simulink model "ass_1"  (R2020a)
settings: Solver=FixedStepAuto  StartTime=0.0  StopTime=10.0  FixedStep=1e-3  RelTol=1e-3  EnableMultiTasking=on
undefined symbols (not defined in the file): D0, D1, D10, D11, D12, D13, D2, D3, D4, D5, D6, D7, D8, D9, PTA0, PTA1, PTA2, PTB23, PTB9, PTC16, PTC17, PTC2, PTC3, PTC4, PTD0, PTD1, PTD2, PTD3
libraries: frdmk64flib x15
settings Model: ExtModeTrigDuration=5  Creator=wxavi  LastModifiedBy=wxavi
settings OptimizationCC: EnhancedBackFolding=on  PassReuseOutputArgsAs=Individual arguments  ZeroExternalMemoryAtStartup=off  ZeroInternalMemoryAtStartup=off  MaxStackSize=64  OptimizeBlockOrder=speed  DifferentSizesBufferReuse=on  OptimizationCustomize=off  EfficientTunableParamExpr=on
settings DebuggingCC: ParameterTunabilityLossMsg=error
settings HardwareCC: ProdBitPerPointer=32  ProdBitPerSizeT=32  ProdBitPerPtrDiffT=32  ProdLargestAtomicInteger=Long  ProdLargestAtomicFloat=Double  ProdWordSize=32  ProdHWDeviceType=ARM Compatible->ARM Cortex
settings SFSimCC: MATLABDynamicMemAlloc=off
settings RTWCC: SystemTargetFile=ert.tlc  HardwareBoard=NXP FRDM-K64F  TemplateMakefile=ert_default_tmf  Toolchain=GNU Tools for ARM Embedded Processors
settings CodeAppCC: ForceParamTrailComments=on  IgnoreCustomStorageClasses=off  OperatorAnnotations=on  SimulinkDataObjDesc=on  SFDataObjDesc=on  InsertBlockDesc=on

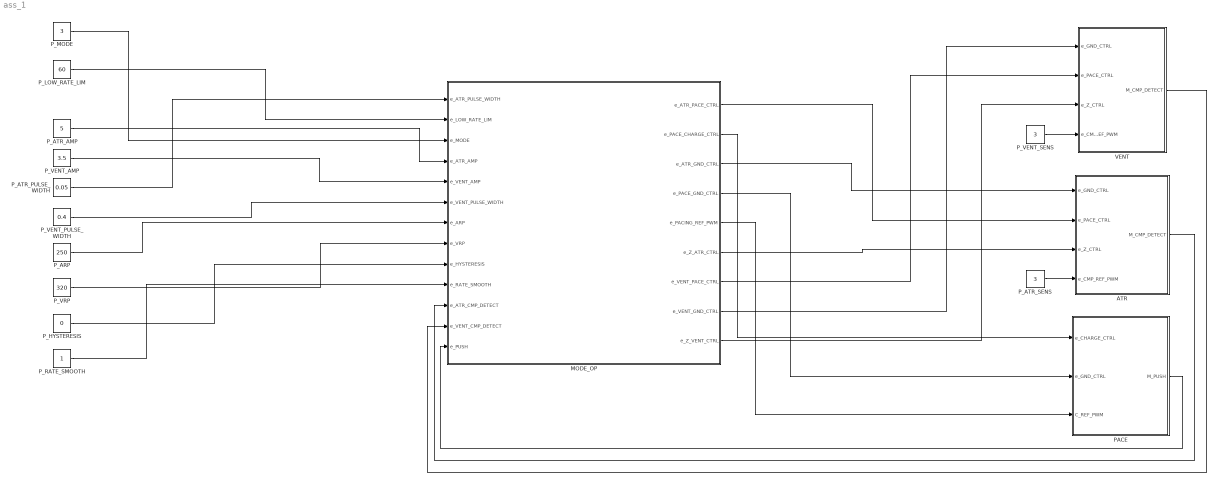
== system ass_1 ==
  ATR : Subsystem
  MODE_OP : Stateflow chart  TreatAsAtomicUnit=on
  PACE : Subsystem
  P_ARP : Constant  Value=250
  P_ATR_AMP : Constant  Value=5
  P_ATR_PULSE_WIDTH : Constant  Value=0.05
  P_ATR_SENS : Constant  Value=3
  P_HYSTERESIS : Constant  Value=0
  P_LOW_RATE_LIM : Constant  Value=60
  P_MODE : Constant  Value=3
  P_RATE_SMOOTH : Constant
  P_VENT_AMP : Constant  Value=3.5
  P_VENT_PULSE_WIDTH : Constant  Value=0.4
  P_VENT_SENS : Constant  Value=3
  P_VRP : Constant  Value=320
  VENT : Subsystem
  wires:
  P_LOW_RATE_LIM/1 -> MODE_OP/2(e_LOW_RATE_LIM)
  P_ATR_AMP/1 -> MODE_OP/4(e_ATR_AMP)
  P_VENT_AMP/1 -> MODE_OP/5(e_VENT_AMP)
  P_ATR_PULSE_WIDTH/1 -> MODE_OP/1(e_ATR_PULSE_WIDTH)
  P_VENT_PULSE_WIDTH/1 -> MODE_OP/6(e_VENT_PULSE_WIDTH)
  P_MODE/1 -> MODE_OP/3(e_MODE)
  P_ATR_SENS/1 -> ATR/4(e_CMP_REF_PWM)
  P_VENT_SENS/1 -> VENT/4(e_CMP_REF_PWM)
  P_ARP/1 -> MODE_OP/7(e_ARP)
  P_VRP/1 -> MODE_OP/8(e_VRP)
  P_HYSTERESIS/1 -> MODE_OP/9(e_HYSTERESIS)
  P_RATE_SMOOTH/1 -> MODE_OP/10(e_RATE_SMOOTH)
  ATR/1(M_CMP_DETECT) -> MODE_OP/11(e_ATR_CMP_DETECT)
  VENT/1(M_CMP_DETECT) -> MODE_OP/12(e_VENT_CMP_DETECT)
  PACE/1(M_PUSH) -> MODE_OP/13(e_PUSH)
  MODE_OP/1(e_ATR_PACE_CTRL) -> ATR/2(e_PACE_CTRL)
  MODE_OP/2(e_PACE_CHARGE_CTRL) -> PACE/1(e_CHARGE_CTRL)
  MODE_OP/3(e_ATR_GND_CTRL) -> ATR/1(e_GND_CTRL)
  MODE_OP/4(e_PACE_GND_CTRL) -> PACE/2(e_GND_CTRL)
  MODE_OP/5(e_PACING_REF_PWM) -> PACE/3(C_REF_PWM)
  MODE_OP/6(e_Z_ATR_CTRL) -> ATR/3(e_Z_CTRL)
  MODE_OP/7(e_VENT_PACE_CTRL) -> VENT/2(e_PACE_CTRL)
  MODE_OP/8(e_VENT_GND_CTRL) -> VENT/1(e_GND_CTRL)
  MODE_OP/9(e_Z_VENT_CTRL) -> VENT/3(e_Z_CTRL)

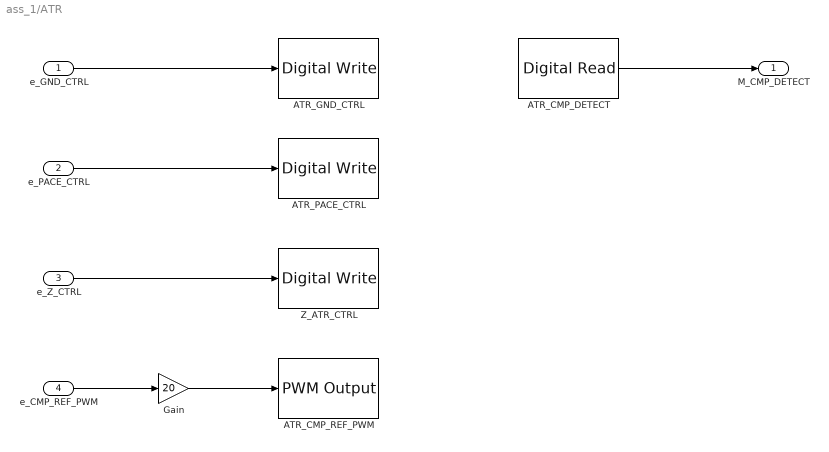
== system ass_1/ATR ==
  e_GND_CTRL : Inport
  e_PACE_CTRL : Inport  Port=2
  e_Z_CTRL : Inport  Port=3
  e_CMP_REF_PWM : Inport  Port=4
  ATR_CMP_DETECT : frdmk64flib/Digital Read  Whichpin=PTC16 (D0)  SampleTime=-1
  ATR_CMP_REF_PWM : frdmk64flib/PWM Output  Whichpin=PTC2 (D6)  InitialFrequency=2000  InitialDutyCycle=0
  ATR_GND_CTRL : frdmk64flib/Digital Write  Whichpin=PTD2 (D11)
  ATR_PACE_CTRL : frdmk64flib/Digital Write  Whichpin=PTA0 (D8)
  Gain : Gain  Gain=20
  Z_ATR_CTRL : frdmk64flib/Digital Write  Whichpin=PTB23 (D4)
  M_CMP_DETECT : Outport
  wires:
  e_Z_CTRL/1 -> Z_ATR_CTRL/1
  e_GND_CTRL/1 -> ATR_GND_CTRL/1
  e_PACE_CTRL/1 -> ATR_PACE_CTRL/1
  e_CMP_REF_PWM/1 -> Gain/1
  ATR_CMP_DETECT/1 -> M_CMP_DETECT/1
  Gain/1 -> ATR_CMP_REF_PWM/1

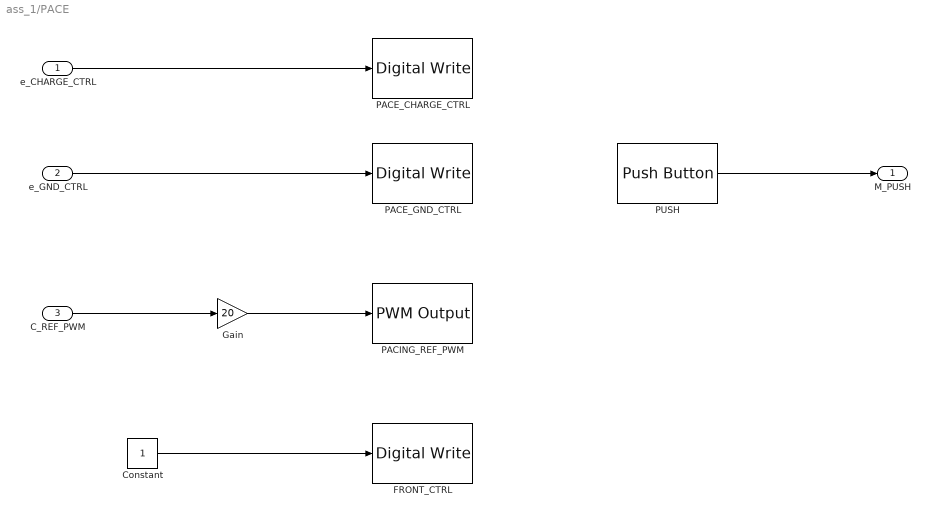
== system ass_1/PACE ==
  e_CHARGE_CTRL : Inport
  e_GND_CTRL : Inport  Port=2
  C_REF_PWM : Inport  Port=3
  Constant : Constant
  FRONT_CTRL : frdmk64flib/Digital Write  Whichpin=PTD1 (D13)
  Gain : Gain  Gain=20
  PACE_CHARGE_CTRL : frdmk64flib/Digital Write  Whichpin=PTB9 (D2)
  PACE_GND_CTRL : frdmk64flib/Digital Write  Whichpin=PTD0 (D10)
  PACING_REF_PWM : frdmk64flib/PWM Output  Whichpin=PTA2 (D5)  InitialFrequency=2000  InitialDutyCycle=0
  PUSH : frdmk64flib/Push Button  Whichswitch=SW2  SampleTime1=-1
  M_PUSH : Outport
  wires:
  Gain/1 -> PACING_REF_PWM/1
  C_REF_PWM/1 -> Gain/1
  e_GND_CTRL/1 -> PACE_GND_CTRL/1
  e_CHARGE_CTRL/1 -> PACE_CHARGE_CTRL/1
  Constant/1 -> FRONT_CTRL/1
  PUSH/1 -> M_PUSH/1

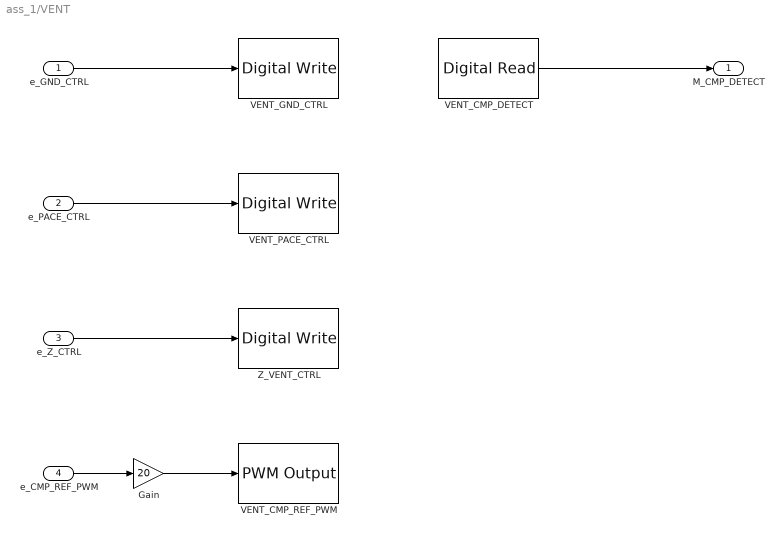
== system ass_1/VENT ==
  e_GND_CTRL : Inport
  e_PACE_CTRL : Inport  Port=2
  e_Z_CTRL : Inport  Port=3
  e_CMP_REF_PWM : Inport  Port=4
  Gain : Gain  Gain=20
  VENT_CMP_DETECT : frdmk64flib/Digital Read  Whichpin=PTC17 (D1)  SampleTime=-1
  VENT_CMP_REF_PWM : frdmk64flib/PWM Output  Whichpin=PTA1 (D3)  InitialFrequency=2000  InitialDutyCycle=0
  VENT_GND_CTRL : frdmk64flib/Digital Write  Whichpin=PTD3 (D12)
  VENT_PACE_CTRL : frdmk64flib/Digital Write  Whichpin=PTC4 (D9)
  Z_VENT_CTRL : frdmk64flib/Digital Write  Whichpin=PTC3 (D7)
  M_CMP_DETECT : Outport
  wires:
  e_GND_CTRL/1 -> VENT_GND_CTRL/1
  e_PACE_CTRL/1 -> VENT_PACE_CTRL/1
  e_Z_CTRL/1 -> Z_VENT_CTRL/1
  e_CMP_REF_PWM/1 -> Gain/1
  VENT_CMP_DETECT/1 -> M_CMP_DETECT/1
  Gain/1 -> VENT_CMP_REF_PWM/1

== stateflow chart ass_1/MODE_OP ==
  state MODE_CHECK
    entry:
    e_PULSE_INT = e_LOW_RATE_LIM/60*1000;
    if (e_MODE == 0 || e_MODE == 3)
    e_PULSE_WIDTH = e_ATR_PULSE_WIDTH;
    e_PULSE_AMP = e_ATR_AMP;
    else
    e_PULSE_WIDTH = e_VENT_PULSE_WIDTH;
    e_PULSE_AMP = e_VENT_AMP;
    end
    e_PACING_REF_PWM = e_PULSE_AMP;
    if (e_MODE == 2 || e_MODE == 3)
    e_PULSE_INT = e_PULSE_INT * e_RATE_SMOOTH + e_HYSTERESIS;
    end
  state AAI_Charge
    entry:
    e_PACE_CHARGE_CTRL = 1;
    e_ATR_GND_CTRL = 1;
    e_ATR_PACE_CTRL = 0;
    e_PACE_GND_CTRL = 1;
    e_VENT_PACE_CTRL = 0;
    e_VENT_GND_CTRL = 0;
    e_Z_ATR_CTRL = 0;
    e_Z_VENT_CTRL = 0;
    e_pushed = 0;
    if(e_PUSH) e_pushed = 1; end
  state AAI_SENSE
    during:
    if(e_PUSH) e_pushed = 1; end
  state AAI_Pace
    entry:
    if (~e_pushed)
    e_PACE_CHARGE_CTRL = 0;
    e_ATR_GND_CTRL = 0;
    e_ATR_PACE_CTRL = 1;
    end
  state VVI_Charge
    entry:
    e_PACE_CHARGE_CTRL = 1;
    e_VENT_GND_CTRL = 1;
    e_VENT_PACE_CTRL = 0;
    e_PACE_GND_CTRL = 1;
    e_ATR_PACE_CTRL = 0;
    e_ATR_GND_CTRL = 0;
    e_Z_ATR_CTRL = 0;
    e_Z_VENT_CTRL = 0;
    e_pushed = 0;
    if(e_PUSH) e_pushed = 1; end
  state VVI_SENSE
    during:
    if(e_PUSH) e_pushed = 1; end
  state VVI_Pace
    entry:
    if (~e_pushed)
    e_PACE_CHARGE_CTRL = 0;
    e_VENT_GND_CTRL = 0;
    e_VENT_PACE_CTRL = 1;
    end
  state AOO_Charge
    entry:
    e_PACE_CHARGE_CTRL = 1;
    e_ATR_GND_CTRL = 1;
    e_ATR_PACE_CTRL = 0;
    e_PACE_GND_CTRL = 1;
    e_VENT_PACE_CTRL = 0;
    e_VENT_GND_CTRL = 0;
    e_Z_ATR_CTRL = 0;
    e_Z_VENT_CTRL = 0;
    e_pushed = 0;
    if(e_PUSH) e_pushed = 1; end
  state AOO_Pace
    entry:
    if (~e_pushed)
    e_PACE_CHARGE_CTRL = 0;
    e_ATR_GND_CTRL = 0;
    e_ATR_PACE_CTRL = 1;
    end
  state VOO_Charge
    entry:
    e_PACE_CHARGE_CTRL = 1;
    e_VENT_GND_CTRL = 1;
    e_VENT_PACE_CTRL = 0;
    e_PACE_GND_CTRL = 1;
    e_ATR_PACE_CTRL = 0;
    e_ATR_GND_CTRL = 0;
    e_Z_ATR_CTRL = 0;
    e_Z_VENT_CTRL = 0;
    e_pushed = 0;
    if(e_PUSH) e_pushed = 1; end
  state VOO_Pace
    entry:
    if (~e_pushed)
    e_PACE_CHARGE_CTRL = 0;
    e_VENT_GND_CTRL = 0;
    e_VENT_PACE_CTRL = 1;
    end
  (default) -> MODE_CHECK
  AAI_Charge -> AAI_SENSE : [after(e_ARP,msec)]
  MODE_CHECK -> AAI_Charge [order 1] : [e_MODE == 2]
  AAI_SENSE -> AAI_Charge [order 2] : [e_ATR_CMP_DETECT]
  AAI_SENSE -> AAI_Pace [order 1] : [after(e_PULSE_INT-e_PULSE_WIDTH-e_ARP,msec) && ~e_ATR_CMP_DETECT]
  AAI_Pace -> AAI_Charge : [after(e_PULSE_WIDTH,msec)]
  MODE_CHECK -> VOO_Charge [order 4] : [e_MODE == 1]
  MODE_CHECK -> AOO_Charge [order 3] : [e_MODE == 0]
  MODE_CHECK -> VVI_Charge [order 2] : [e_MODE == 3]
  VVI_Charge -> VVI_SENSE : [after(e_VRP,msec)]
  VVI_SENSE -> VVI_Charge [order 1] : [e_VENT_CMP_DETECT]
  VVI_SENSE -> VVI_Pace [order 2] : [after(e_PULSE_INT - e_PULSE_WIDTH-e_VRP,msec) && ~e_VENT_CMP_DETECT]
  VVI_Pace -> VVI_Charge : [after(e_PULSE_WIDTH,msec)]
  AOO_Charge -> AOO_Pace : [[[after(e_PULSE_INT - e_PULSE_WIDTH,msec)]]]
  AOO_Pace -> AOO_Charge : [after(e_PULSE_WIDTH,msec)]
  VOO_Charge -> VOO_Pace : [[after(e_PULSE_INT - e_PULSE_WIDTH,msec)]]
  VOO_Pace -> VOO_Charge : [after(e_PULSE_WIDTH,msec)]
  data: e_ATR_PULSE_WIDTH input double; e_ATR_PACE_CTRL output int16; e_PACE_CHARGE_CTRL output int16; e_ATR_GND_CTRL output int16; e_LOW_RATE_LIM input double; e_MODE input double; e_ATR_AMP input double; e_VENT_AMP input double; e_VENT_PULSE_WIDTH input double; e_PACE_GND_CTRL output int16; e_PACING_REF_PWM output double; e_Z_ATR_CTRL output int16; e_VENT_PACE_CTRL output int16; e_VENT_GND_CTRL output int16; e_Z_VENT_CTRL output int16; e_ARP input double; e_VRP input double; e_HYSTERESIS input double; e_RATE_SMOOTH input double; e_ATR_CMP_DETECT input boolean; e_VENT_CMP_DETECT input boolean; e_PUSH input boolean; e_pushed local int16; e_PULSE_WIDTH local double; e_PULSE_INT local double; e_PULSE_AMP local double
